simulink model "Example"  (R2018a)
settings: Solver=ode45  StartTime=0.0  StopTime=10.0  RelTol=1e-3
undefined symbols (not defined in the file or in its folder): k
settings Model: Creator=rattle  LastModifiedBy=rattle

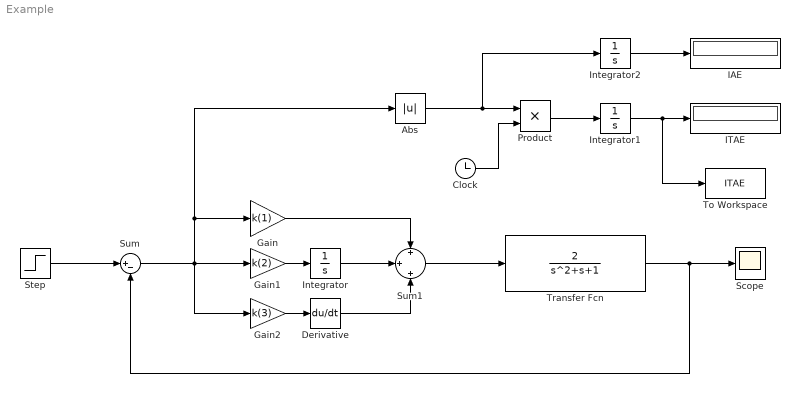
== system Example ==
  Abs : Abs
  Clock : Clock
  Derivative : Derivative
  Gain : Gain  Gain=k(1)
  Gain1 : Gain  Gain=k(2)
  Gain2 : Gain  Gain=k(3)
  IAE : Display
  ITAE : Display
  Integrator : Integrator
  Integrator1 : Integrator
  Integrator2 : Integrator
  Product : Product
  Scope : Scope
  Step : Step  SampleTime=0
  Sum : Sum  Inputs=|+-
  Sum1 : Sum  Inputs=+|+|+
  To Workspace : ToWorkspace  VariableName=ITAE  SampleTime=-1
  Transfer Fcn : TransferFcn  Numerator=[2]  Denominator=[1 1 1]
  wires:
  Transfer Fcn/1 -> Scope/1, Sum/2
  Gain2/1 -> Derivative/1
  Gain1/1 -> Integrator/1
  Sum/1 -> Gain2/1, Abs/1, Gain/1, Gain1/1
  Sum1/1 -> Transfer Fcn/1
  Integrator/1 -> Sum1/2
  Derivative/1 -> Sum1/3
  Gain/1 -> Sum1/1
  Step/1 -> Sum/1
  Abs/1 -> Integrator2/1, Product/1
  Clock/1 -> Product/2
  Product/1 -> Integrator1/1
  Integrator1/1 -> To Workspace/1, ITAE/1
  Integrator2/1 -> IAE/1
